simulink model "HIL_Climber_HVAC_Control_V5"  (R2021a)
settings: Solver=VariableStepAuto  StartTime=0.0  StopTime=10.0  RelTol=1e-3
settings Model: Creator=leela  LastModifiedBy=prasad

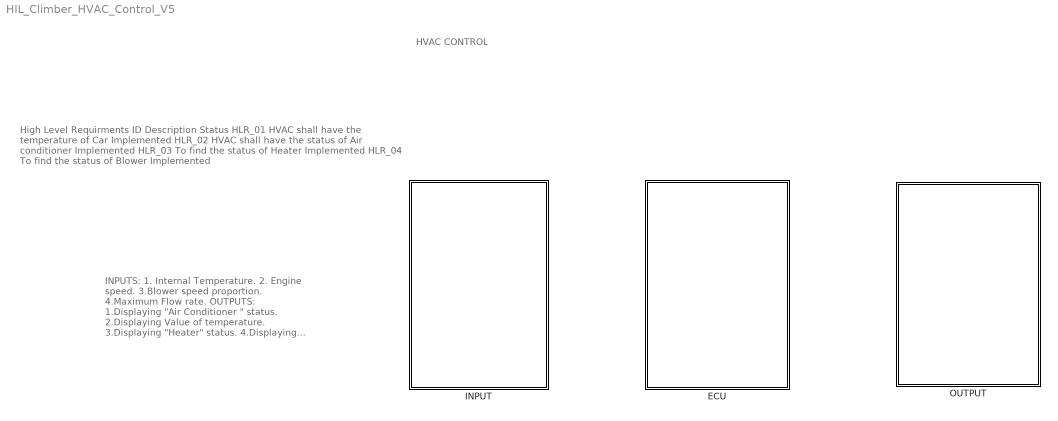
== system HIL_Climber_HVAC_Control_V5 ==
  note: INPUTS:
      | 1. Internal Temperature.
      | 2. Engine speed.
      | 3.Blower speed proportion.
      | 4.Maximum Flow rate.
      |
      | OUTPUTS:
      | 1.Displaying "Air Conditioner " status.
      | 2.Displaying Value of temperature.
      | 3.Displaying "Heater" status.
      | 4.Displaying "Blower" status.
  note: High Level Requirments
      |
      | ID
      | Description
      | Status
      |
      | HLR_01
      | HVAC shall have the temperature of Car
      | Implemented
      |
      | HLR_02
      | HVAC shall have the status of Air conditioner
      | Implemented
      |
      | HLR_03
      | To find the status of Heater
      | Implemented
      |
      | HLR_04
      | To find the status of Blower
      | Implemented
  note: HVAC CONTROL
  ECU : Subsystem  ReferencedSubsystem=HVAC_ECU
  INPUT : Subsystem
  OUTPUT : Subsystem

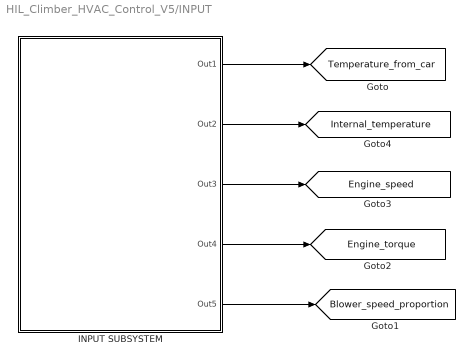
== system HIL_Climber_HVAC_Control_V5/INPUT ==
  INPUT SUBSYSTEM : Subsystem
  tag scope: Blower_speed_proportion=global, Engine_speed=global, Engine_torque=global, Internal_temperature=global, Temperature_from_car=global
  wires:
  INPUT SUBSYSTEM/3(Out3) -> [Engine_speed]
  INPUT SUBSYSTEM/5(Out5) -> [Blower_speed_proportion]
  INPUT SUBSYSTEM/1(Out1) -> [Temperature_from_car]
  INPUT SUBSYSTEM/2(Out2) -> [Internal_temperature]
  INPUT SUBSYSTEM/4(Out4) -> [Engine_torque]

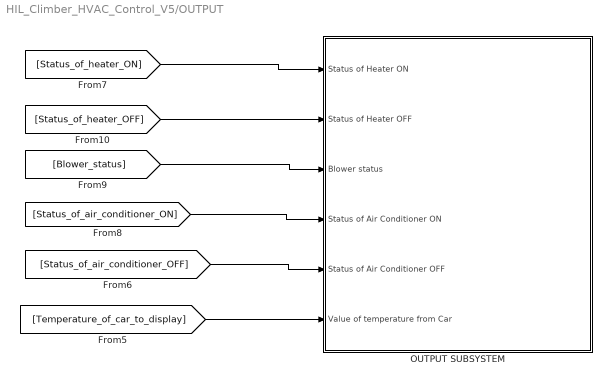
== system HIL_Climber_HVAC_Control_V5/OUTPUT ==
  OUTPUT SUBSYSTEM : Subsystem
  wires:
  [Status_of_heater_ON] -> OUTPUT SUBSYSTEM/1(Status of Heater ON)
  [Status_of_air_conditioner_ON] -> OUTPUT SUBSYSTEM/4(Status of Air Conditioner ON)
  [Blower_status] -> OUTPUT SUBSYSTEM/3(Blower status)
  [Temperature_of_car_to_display] -> OUTPUT SUBSYSTEM/6(Value of temperature from Car)
  [Status_of_heater_OFF] -> OUTPUT SUBSYSTEM/2(Status of Heater OFF)
  [Status_of_air_conditioner_OFF] -> OUTPUT SUBSYSTEM/5(Status of Air Conditioner OFF)

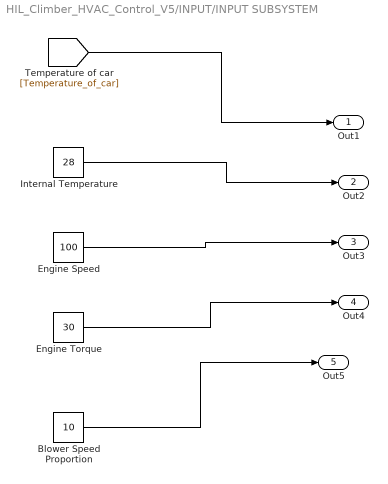
== system HIL_Climber_HVAC_Control_V5/INPUT/INPUT SUBSYSTEM ==
  Blower Speed Proportion : Constant  Value=10
  Engine Speed : Constant  Value=100
  Engine Torque : Constant  Value=30
  Internal Temperature : Constant  Value=28
  Out1 : Outport
  Out2 : Outport  Port=2
  Out3 : Outport  Port=3
  Out4 : Outport  Port=4
  Out5 : Outport  Port=5
  wires:
  Engine Speed/1 -> Out3/1
  Blower Speed Proportion/1 -> Out5/1
  Internal Temperature/1 -> Out2/1
  Engine Torque/1 -> Out4/1
  [Temperature_of_car] -> Out1/1

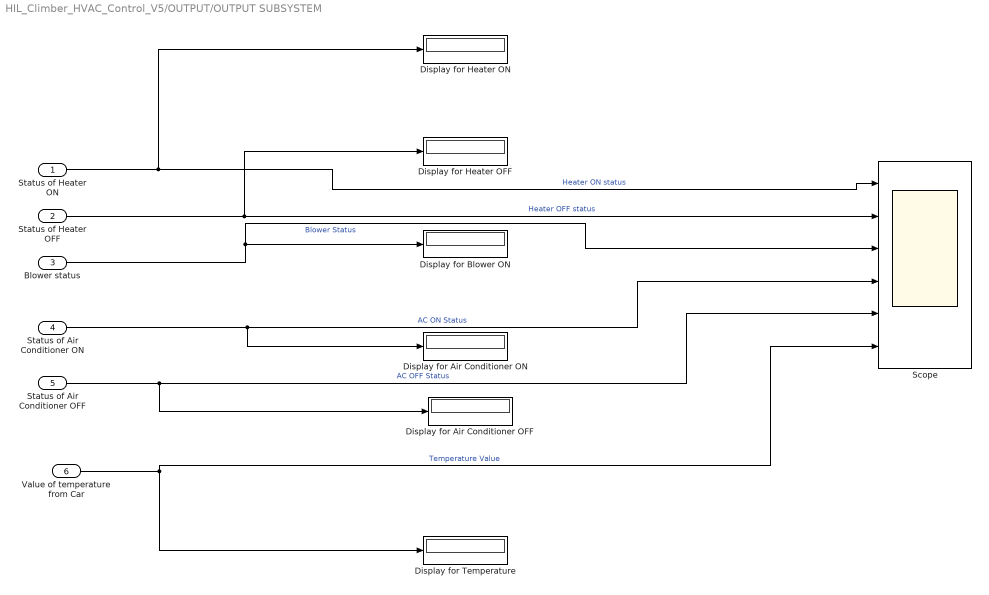
== system HIL_Climber_HVAC_Control_V5/OUTPUT/OUTPUT SUBSYSTEM ==
  Status of Heater ON : Inport
  Status of Heater OFF : Inport  Port=2
  Blower status : Inport  Port=3
  Status of Air Conditioner ON : Inport  Port=4
  Status of Air Conditioner OFF : Inport  Port=5
  Value of temperature from Car : Inport  Port=6
  Display for Air Conditioner OFF : Display
  Display for Air Conditioner ON : Display
  Display for Blower ON : Display
  Display for Heater OFF : Display
  Display for Heater ON : Display
  Display for Temperature : Display
  Scope : Scope  NumInputPorts=6
  wires:
  Status of Air Conditioner ON/1 -> Scope/4, Display for Air Conditioner ON/1  "AC ON Status"
  Blower status/1 -> Scope/3, Display for Blower ON/1  "Blower Status"
  Status of Heater ON/1 -> Scope/1, Display for Heater ON/1  "Heater ON status"
  Value of temperature from Car/1 -> Scope/6, Display for Temperature/1  "Temperature Value"
  Status of Heater OFF/1 -> Scope/2, Display for Heater OFF/1  "Heater OFF status"
  Status of Air Conditioner OFF/1 -> Scope/5, Display for Air Conditioner OFF/1  "AC OFF Status"
